simulink library "simlib_vpc_basic"  (R2022a)
settings: Solver=VariableStepAuto  StartTime=0.0  StopTime=10.0  RelTol=1e-3
undefined symbols (not defined in the file or in its folder): __PRM__SERIALIZED__DATA__, Ad, Camera, Pinhole, RBM, RRBM, VMO, VPC
libraries: $bdroot x10, simlib_vpc_coremath x5
(part 2 of 2)

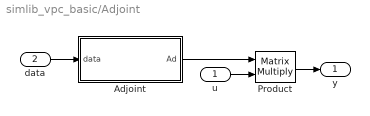
== system simlib_vpc_basic/Adjoint ==
  u : Inport
  data : Inport  Port=2
  Adjoint : MATLAB Function  TreatAsAtomicUnit=on
  Product : Product  Multiplication=Matrix(*)
  y : Outport
  wires:
  u/1 -> Product/2
  Adjoint/1(Ad) -> Product/1
  data/1 -> Adjoint/1(data)
  Product/1 -> y/1

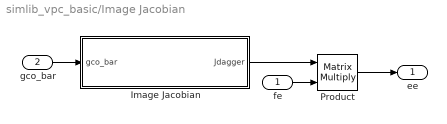
== system simlib_vpc_basic/Image Jacobian ==
  fe : Inport
  gco_bar : Inport  Port=2
  Image Jacobian : MATLAB Function  TreatAsAtomicUnit=on
  Product : Product  Multiplication=Matrix(*)
  ee : Outport
  wires:
  fe/1 -> Product/2
  Image Jacobian/1(Jdagger) -> Product/1
  gco_bar/1 -> Image Jacobian/1(gco_bar)
  Product/1 -> ee/1

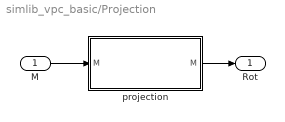
== system simlib_vpc_basic/Projection ==
  M : Inport
  projection : MATLAB Function  TreatAsAtomicUnit=on
  Rot : Outport
  wires:
  M/1 -> projection/1("M ")
  projection/1(M) -> Rot/1

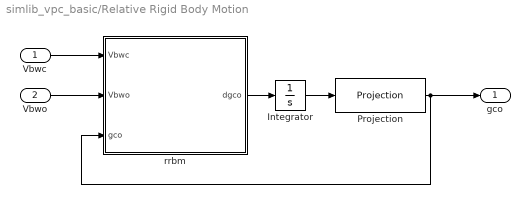
== system simlib_vpc_basic/Relative Rigid Body Motion ==
  Vbwc : Inport
  Vbwo : Inport  Port=2
  Integrator : Integrator  InitialCondition=gco0
  Projection : $bdroot/Projection  projectiontype=averaging  inputtype=pose
  rrbm : MATLAB Function  TreatAsAtomicUnit=on
  gco : Outport
  wires:
  Vbwc/1 -> rrbm/1(Vbwc)
  rrbm/1(dgco) -> Integrator/1
  Vbwo/1 -> rrbm/2(Vbwo)
  Integrator/1 -> Projection/1
  Projection/1 -> gco/1, rrbm/3(gco)

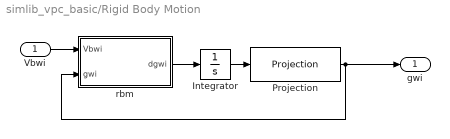
== system simlib_vpc_basic/Rigid Body Motion ==
  Vbwi : Inport
  Integrator : Integrator  InitialCondition=g0  ContinuousStateAttributes='pose'
  Projection : $bdroot/Projection  projectiontype=averaging  inputtype=pose
  rbm : MATLAB Function  TreatAsAtomicUnit=on
  gwi : Outport
  wires:
  rbm/1(dgwi) -> Integrator/1
  Vbwi/1 -> rbm/1(Vbwi)
  Integrator/1 -> Projection/1
  Projection/1 -> gwi/1, rbm/2(gwi)

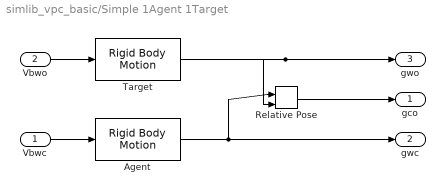
== system simlib_vpc_basic/Simple 1Agent 1Target ==
  Vbwc : Inport
  Vbwo : Inport  Port=2
  Agent : $bdroot/Rigid Body Motion  rbmtype=agent  agentnumber=1  projection=on  show_dg=off  g0=gwc0
  Relative Pose : simlib_vpc_coremath/Relative Pose
      settings: SourceProductName=VPC Library
  Target : $bdroot/Rigid Body Motion  rbmtype=target  agentnumber=1  projection=on  show_dg=off  g0=gwo0
  gco : Outport
  gwc : Outport  Port=2
  gwo : Outport  Port=3
  wires:
  Vbwc/1 -> Agent/1
  Relative Pose/1 -> gco/1
  Target/1 -> Relative Pose/2, gwo/1
  Vbwo/1 -> Target/1
  Agent/1 -> Relative Pose/1, gwc/1

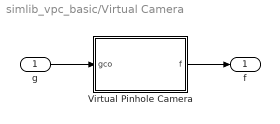
== system simlib_vpc_basic/Virtual Camera ==
  g : Inport
  Virtual Pinhole Camera : MATLAB Function  TreatAsAtomicUnit=on
  f : Outport
  wires:
  Virtual Pinhole Camera/1(f) -> f/1
  g/1 -> Virtual Pinhole Camera/1(gco)

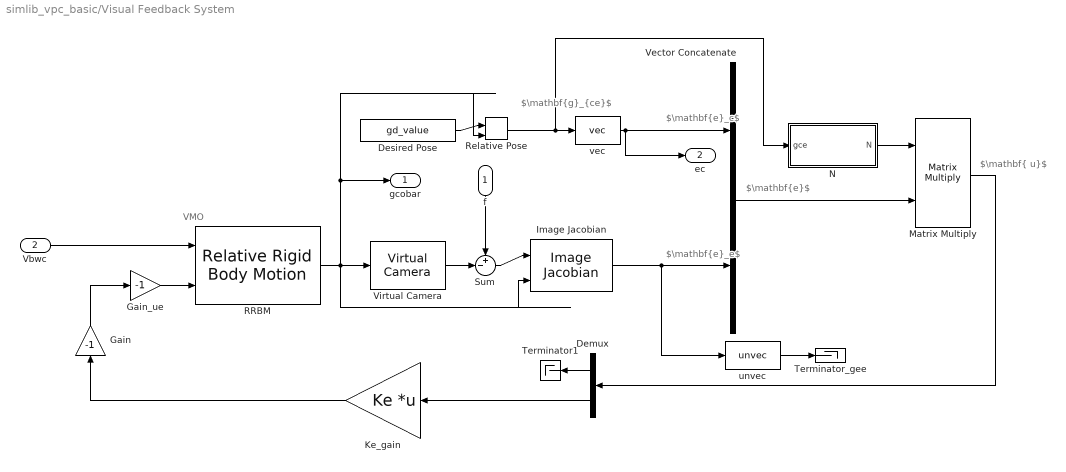
== system simlib_vpc_basic/Visual Feedback System ==
  note: VMO
  note: $\mathbf{e}_c$
  note: $\mathbf{e}_e$
  note: $\mathbf{e}$
  note: $\mathbf{g}_{ce}$
  note: $\mathbf{\nu}$
  f : Inport
  Vbwc : Inport  Port=2
  Demux : Demux  Outputs=2
  Desired Pose : Constant  Value=gd_value
  Gain : Gain  Gain=-1
  Gain_ue : Gain  Gain=-1
  Image Jacobian : $bdroot/Image Jacobian  po=fo  lambda=lambda
  Ke_gain : Gain  Gain=Ke  Multiplication=Matrix(K*u) (u vector)
  Matrix Multiply : Product  Multiplication=Matrix(*)
  N : MATLAB Function  TreatAsAtomicUnit=on
  RRBM : $bdroot/Relative Rigid Body Motion  gco0=gcobar0  projection=on  show_dgco=off
  Relative Pose : simlib_vpc_coremath/Relative Pose
      settings: SourceProductName=VPC Library
  Sum : Sum  Inputs=+-|
  Terminator1 : Terminator
  Terminator_gee : Terminator
  Vector Concatenate : Concatenate
  Virtual Camera : $bdroot/Virtual Camera  camtype=Pinhole  po=fo  lambda=lambda
  unvec : simlib_vpc_coremath/unvec
      settings: SourceProductName=VPC Library
  vec : simlib_vpc_coremath/vec
      settings: SourceProductName=VPC Library
  gcobar : Outport
  ec : Outport  Port=2
  wires:
  Relative Pose/1 -> N/1(gce), vec/1
  Vector Concatenate/1 -> Matrix Multiply/2
  Matrix Multiply/1 -> Demux/1
  N/1(N) -> Matrix Multiply/1
  vec/1 -> Vector Concatenate/1, ec/1
  Image Jacobian/1 -> unvec/1, Vector Concatenate/2
  RRBM/1 -> Relative Pose/2, gcobar/1, Image Jacobian/2, Virtual Camera/1
  Vbwc/1 -> RRBM/1
  Sum/1 -> Image Jacobian/1
  f/1 -> Sum/1
  Gain_ue/1 -> RRBM/2
  Virtual Camera/1 -> Sum/2
  Demux/1 -> Terminator1/1
  Demux/2 -> Ke_gain/1
  Ke_gain/1 -> Gain/1
  Gain/1 -> Gain_ue/1
  Desired Pose/1 -> Relative Pose/1
  unvec/1 -> Terminator_gee/1

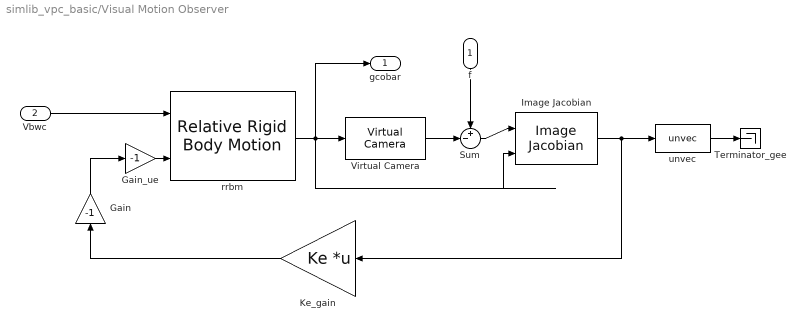
== system simlib_vpc_basic/Visual Motion Observer ==
  f : Inport
  Vbwc : Inport  Port=2
  Gain : Gain  Gain=-1
  Gain_ue : Gain  Gain=-1
  Image Jacobian : $bdroot/Image Jacobian  po=fo  lambda=lambda
  Ke_gain : Gain  Gain=Ke  Multiplication=Matrix(K*u) (u vector)
  Sum : Sum  Inputs=+-|
  Terminator_gee : Terminator
  Virtual Camera : $bdroot/Virtual Camera  camtype=Pinhole  po=fo  lambda=lambda
  rrbm : $bdroot/Relative Rigid Body Motion  gco0=gcobar0  projection=on  show_dgco=off
  unvec : simlib_vpc_coremath/unvec
      settings: SourceProductName=VPC Library
  gcobar : Outport
  wires:
  Virtual Camera/1 -> Sum/2
  rrbm/1 -> gcobar/1, Image Jacobian/2, Virtual Camera/1
  Sum/1 -> Image Jacobian/1
  f/1 -> Sum/1
  Vbwc/1 -> rrbm/1
  Gain_ue/1 -> rrbm/2
  Image Jacobian/1 -> Ke_gain/1, unvec/1
  Ke_gain/1 -> Gain/1
  Gain/1 -> Gain_ue/1
  unvec/1 -> Terminator_gee/1

== matlab function simlib_vpc_basic/Image Jacobian/Image Jacobian ==
  data: Jdagger output; gco_bar input size=[4,4]; lambda parameter size=1; po parameter
function Jdagger = slx_imageJacobian(gco_bar, lambda, po) %#codegen
% Function Wrapper
%
% Editor:
%   OMAINSKA Marco - Doctoral Student, Cybernetics
%       <marcoomainska@g.ecc.u-tokyo.ac.jp>
% Review:
%   YAMAUCHI Junya - Assistant Professor
%       <junya_yamauchi@ipc.i.u-tokyo.ac.jp>
%
% Property of: Fujita-Yamauchi Lab, University of Tokyo, 2021
% e-mail: marcoomainska@g.ecc.u-tokyo.ac.jp
% Website: https://www.scl.ipc.i.u-tokyo.ac.jp
% March 2021, Last modified: 2021-MAR-08
%
%------------- BEGIN CODE --------------

% "inverseImageJacobian" is a MATLAB function on the MATLAB path
Jdagger = inverseImageJacobian(gco_bar, lambda, po);

%-------------- END CODE ---------------
end

== matlab function simlib_vpc_basic/Virtual Camera/Virtual Pinhole Camera ==
  data: gco input size=[4,4]; f output; lambda parameter size=1; po parameter; camtype parameter
function f = slx_vcamera(gco, lambda, po, camtype) %#codegen
% Function Wrapper
%
% Editor:
%   OMAINSKA Marco - Doctoral Student, Cybernetics
%       <marcoomainska@g.ecc.u-tokyo.ac.jp>
% Review:
%   YAMAUCHI Junya - Assistant Professor
%       <junya_yamauchi@ipc.i.u-tokyo.ac.jp>
%
% Property of: Fujita-Yamauchi Lab, University of Tokyo, 2021
% e-mail: marcoomainska@g.ecc.u-tokyo.ac.jp
% Website: https://www.scl.ipc.i.u-tokyo.ac.jp
% March 2021, Last modified: 2021-MAR-08
%
%------------- BEGIN CODE --------------

% "vcamera" is a MATLAB function on the MATLAB path
switch camtype
    case 1 %'Pinhole'
        f = vcamera(gco, lambda, po, 'Pinhole');
end

%-------------- END CODE ---------------
end

== matlab function simlib_vpc_basic/Adjoint/Adjoint ==
  data: Ad output size=[6,6]; data input; adjointtype parameter size=1
function Ad = slx_adjoint(data, adjointtype) %#codegen
% Function Wrapper
%
% Editor:
%   OMAINSKA Marco - Doctoral Student, Cybernetics
%       <marcoomainska@g.ecc.u-tokyo.ac.jp>
% Review:
%   YAMAUCHI Junya - Assistant Professor
%       <junya_yamauchi@ipc.i.u-tokyo.ac.jp>
%
% Property of: Fujita-Yamauchi Lab, University of Tokyo, 2021
% e-mail: marcoomainska@g.ecc.u-tokyo.ac.jp
% Website: https://www.scl.ipc.i.u-tokyo.ac.jp
% March 2021, Last modified: 2021-MAR-08
%
%------------- BEGIN CODE --------------

% "adjoint" is a MATLAB function on the MATLAB path
switch adjointtype
    case 1 %'pose'
        Ad = adjoint(data, 'pose');
    case 2 %'position'
        Ad = adjoint(data, 'position');
    case 3 %'orientation'
        Ad = adjoint(data, 'orientation');
    otherwise
        warning('Adjoint type not supported');
end

%------------- END CODE --------------
end

== matlab function simlib_vpc_basic/Rigid Body Motion/rbm ==
  data: Vbwi input size=6; dgwi output size=[4,4]; gwi input size=[4,4]
function dgwi = slx_rbm(Vbwi,gwi) %#codegen
% Function Wrapper
%
% Editor:
%   OMAINSKA Marco - Doctoral Student, Cybernetics
%       <marcoomainska@g.ecc.u-tokyo.ac.jp>
% Review:
%   YAMAUCHI Junya - Assistant Professor
%       <junya_yamauchi@ipc.i.u-tokyo.ac.jp>
%
% Property of: Fujita-Yamauchi Lab, University of Tokyo, 2021
% e-mail: marcoomainska@g.ecc.u-tokyo.ac.jp
% Website: https://www.scl.ipc.i.u-tokyo.ac.jp
% March 2021, Last modified: 2021-MAR-08
%
%------------- BEGIN CODE --------------

% "rbm" is a MATLAB function on the MATLAB path
dgwi = rbm(Vbwi, gwi);

%------------- END CODE --------------
end

== matlab function simlib_vpc_basic/Projection/projection ==
  data: M input; M output; projectiontype parameter; inputtype parameter
function M = slx_projectionSO3(M, projectiontype, inputtype) %#codegen
% Function Wrapper
%
% Editor:
%   OMAINSKA Marco - Doctoral Student, Cybernetics
%       <marcoomainska@g.ecc.u-tokyo.ac.jp>
% Review:
%   YAMAUCHI Junya - Assistant Professor
%       <junya_yamauchi@ipc.i.u-tokyo.ac.jp>
%
% Property of: Fujita-Yamauchi Lab, University of Tokyo, 2021
% e-mail: marcoomainska@g.ecc.u-tokyo.ac.jp
% Website: https://www.scl.ipc.i.u-tokyo.ac.jp
% March 2021, Last modified: 2021-MAR-08
%
%------------- BEGIN CODE --------------

% "projectionSO3" is a MATLAB function on the MATLAB path
switch inputtype
    case 1 %'rotation matrix'
        M = projectionSO3(M);
    case 2 %'pose'
        [M_,p] = splitpose(M);
        M_     = projectionSO3(M_);
        M      = mergepose(M_,p);
    otherwise
        error('Unknown input type!')
end

%-------------- END CODE ---------------
end

== matlab function simlib_vpc_basic/Relative Rigid Body Motion/rrbm ==
  data: Vbwc input size=6; Vbwo input size=6; dgco output size=[4,4]; gco input size=[4,4]
function dgco = slx_rrbm(Vbwc,Vbwo,gco) %#codegen
% Function Wrapper
%
% Editor:
%   OMAINSKA Marco - Doctoral Student, Cybernetics
%       <marcoomainska@g.ecc.u-tokyo.ac.jp>
% Review:
%   YAMAUCHI Junya - Assistant Professor
%       <junya_yamauchi@ipc.i.u-tokyo.ac.jp>
%
% Property of: Fujita-Yamauchi Lab, University of Tokyo, 2021
% e-mail: marcoomainska@g.ecc.u-tokyo.ac.jp
% Website: https://www.scl.ipc.i.u-tokyo.ac.jp
% March 2021, Last modified: 2021-MAR-08
%
%------------- BEGIN CODE --------------

% "rrbm" is a MATLAB function on the MATLAB path
dgco = rrbm(Vbwc, Vbwo, gco);

%------------- END CODE --------------
end

== matlab function simlib_vpc_basic/Visual Feedback System/N ==
  data: gce input size=[4,4]; N output size=[12,12]
function N = slx_NAdj(gce) %#codegen
% Function Wrapper
%
% Editor:
%   OMAINSKA Marco - Doctoral Student, Cybernetics
%       <marcoomainska@g.ecc.u-tokyo.ac.jp>
% Review:
%   YAMAUCHI Junya - Assistant Professor
%       <junya_yamauchi@ipc.i.u-tokyo.ac.jp>
%
% Property of: Fujita-Yamauchi Lab, University of Tokyo, 2021
% e-mail: marcoomainska@g.ecc.u-tokyo.ac.jp
% Website: https://www.scl.ipc.i.u-tokyo.ac.jp
% March 2021, Last modified: 2021-MAR-08
%
%------------- BEGIN CODE --------------

% "NAdj" is a MATLAB function on the MATLAB path
N = NAdj(gce);

%------------- END CODE --------------
end
